simulink model "DC_motor_PIDAW"  (R2015b)
settings: Solver=VariableStepAuto  StartTime=0.0  StopTime=10  MaxStep=1e-2  RelTol=1e-3
settings Model: Creator=mgreiff  LastModifiedBy=mgreiff
settings DebuggingCC: AlgebraicLoopMsg=none

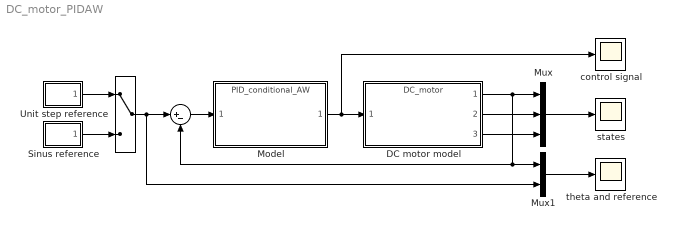
== system DC_motor_PIDAW ==
  " " : Sum  Inputs=|+-
  "   " : ManualSwitch
  DC motor model : ModelReference  ModelNameDialog=DC_motor.slx  SimulationMode=Normal  ModelReferenceVersion=1.8  CopyOfModelName=DC_motor.slx
  Model : ModelReference  ModelNameDialog=PID_conditional_AW.slx  SimulationMode=Normal  ModelReferenceVersion=1.3  CopyOfModelName=PID_conditional_AW.slx
  Mux : Mux  Inputs=3
  Mux1 : Mux  Inputs=2
  Sinus reference : Subsystem
  Unit step reference : Subsystem
  control signal : Scope
  states : Scope
  theta and reference : Scope
  wires:
  DC motor model/1 -> " "/2, Mux1/1, Mux/1
  DC motor model/2 -> Mux/2
  DC motor model/3 -> Mux/3
  Mux/1 -> states/1
  Unit step reference/1(voltage) -> "   "/1
  Sinus reference/1(voltage) -> "   "/2
  Model/1 -> control signal/1, DC motor model/1
  "   "/1 -> Mux1/2, " "/1
  " "/1 -> Model/1
  Mux1/1 -> theta and reference/1

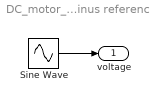
== system DC_motor_PIDAW/Sinus reference ==
  Sine Wave : Sin  Frequency=2*pi/10  SampleTime=0
  voltage : Outport
  wires:
  Sine Wave/1 -> voltage/1

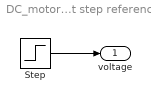
== system DC_motor_PIDAW/Unit step reference ==
  Step : Step  Time=0  SampleTime=0
  voltage : Outport
  wires:
  Step/1 -> voltage/1
